simulink model "QuarterCarModelVer1"  (R2024b)
settings: Solver=VariableStepAuto  StartTime=0.0  StopTime=10  MaxStep=0.0001  RelTol=1e-3
model workspace (MAT data in the model file):
  bs = 1500
  bt = 10
  f = 1
  ks = 20000
  kt = 190000
  ms = 400
  mu = 48
settings Model: Creator=khalidwaleed  LastModifiedBy=khalidwaleed

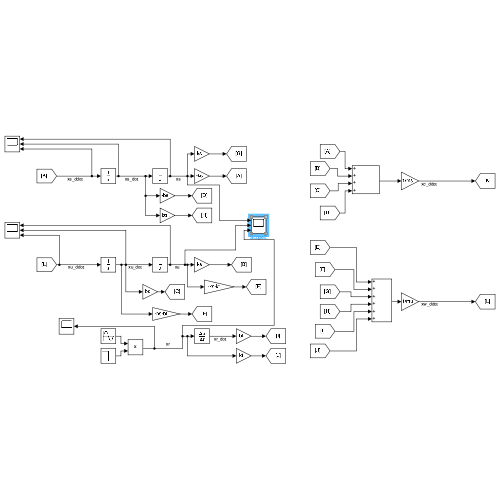
[thumbnail: Simulink's stored preview of the top-level diagram]
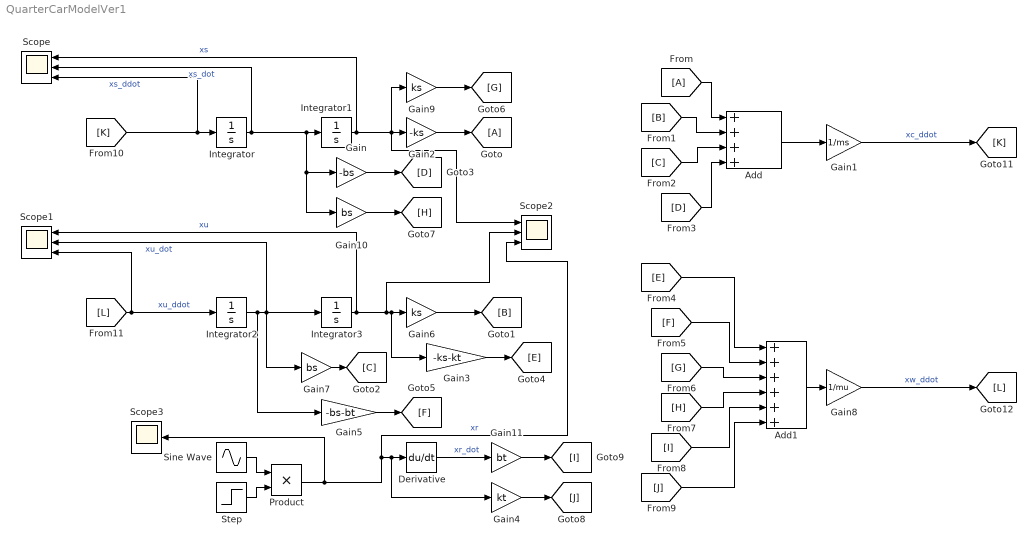
== system QuarterCarModelVer1 ==
  Add : Sum  Inputs=++++
  Add1 : Sum  Inputs=++++++
  Derivative : Derivative
  From : From
  Gain : Gain  Gain=-bs
  Gain1 : Gain  Gain=1/ms
  Gain10 : Gain  Gain=bs
  Gain11 : Gain  Gain=bt
  Gain2 : Gain  Gain=-ks
  Gain3 : Gain  Gain=-ks-kt
  Gain4 : Gain  Gain=kt
  Gain5 : Gain  Gain=-bs-bt
  Gain6 : Gain  Gain=ks
  Gain7 : Gain  Gain=bs
  Gain8 : Gain  Gain=1/mu
  Gain9 : Gain  Gain=ks
  Goto : Goto
  Integrator{,1..3} (4 alike) : Integrator
  Product : Product
  Scope : Scope  NumInputPorts=3
  Scope1 : Scope  NumInputPorts=3
  Scope2 : Scope  NumInputPorts=3
  Scope3 : Scope
  Sine Wave : Sin  Amplitude=0.08  SampleTime=0
  Step : Step  Time=pi  Before=1  After=0  SampleTime=0
  wires:
  Integrator2/1 -> Scope1/2, Gain7/1, Integrator3/1, Gain5/1  "xu_dot"
  Integrator/1 -> Scope/2, Gain10/1, Gain/1, Integrator1/1  "xs_dot"
  Gain1/1 -> [K]  "xc_ddot"
  Integrator1/1 -> Scope/1, Gain9/1, Scope2/1, Gain2/1  "xs"
  Integrator3/1 -> Scope1/1, Gain3/1, Gain6/1, Scope2/2  "xu"
  Add/1 -> Gain1/1
  Add1/1 -> Gain8/1
  Product/1 -> Scope3/1, Scope2/3, Gain4/1, Derivative/1  "xr"
  Derivative/1 -> Gain11/1  "xr_dot"
  Gain2/1 -> Goto/1
  From/1 -> Add/1
  Gain6/1 -> [B]
  [B] -> Add/2
  Gain7/1 -> [C]
  [C] -> Add/3
  Gain/1 -> [D]
  [D] -> Add/4
  Gain3/1 -> [E]
  [E] -> Add1/1
  Gain5/1 -> [F]
  [F] -> Add1/2
  Gain9/1 -> [G]
  [G] -> Add1/3
  Gain10/1 -> [H]
  [H] -> Add1/4
  [I] -> Add1/5
  [J] -> Add1/6
  Gain11/1 -> [I]
  Gain4/1 -> [J]
  [K] -> Scope/3, Integrator/1  "xs_ddot"
  [L] -> Scope1/3, Integrator2/1  "xu_ddot"
  Gain8/1 -> [L]  "xw_ddot"
  Sine Wave/1 -> Product/1
  Step/1 -> Product/2
